simulink model "untitled"  (R2021a)
settings: Solver=VariableStepAuto  StartTime=0.0  StopTime=10  FixedStep=0.1  RelTol=0.001
libraries: simulink x1
settings Model: Creator=VTX  LastModifiedBy=VTX

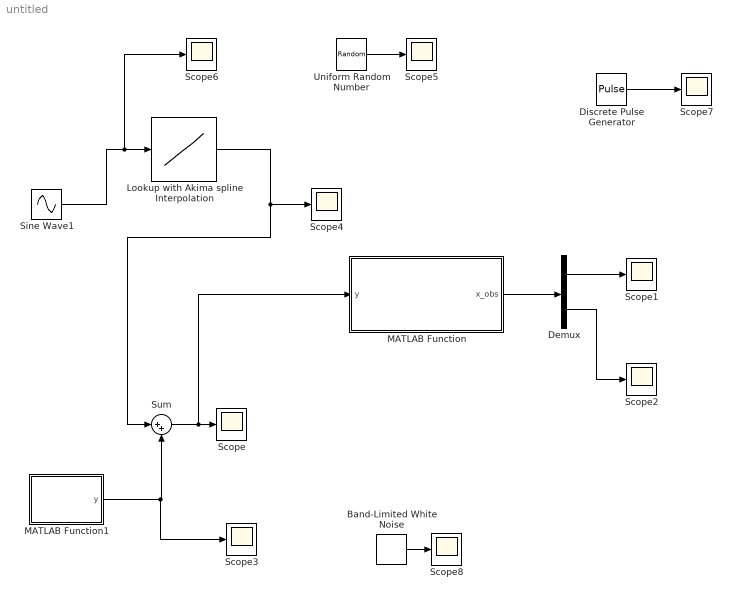
== system untitled ==
  Band-Limited White Noise : simulink/Sources/Band-Limited White Noise  Cov=[0.1]  Ts=0.1  seed=[23341]
  Demux : Demux  Outputs=2
  Discrete Pulse Generator : DiscretePulseGenerator  Period=10  PulseWidth=5  SampleTime=2
  Lookup with Akima spline Interpolation : Lookup_n-D  NumberOfTableDimensions=1  BreakpointsForDimension1=[-5:5]  Table=tanh([-5:5])  InterpMethod=Akima spline  InternalRulePriority=Speed  RndMeth=Simplest  InputSameDT=on
  MATLAB Function : MATLAB Function  TreatAsAtomicUnit=on
  MATLAB Function1 : MATLAB Function  TreatAsAtomicUnit=on
  Scope{,1..8} (9 alike) : Scope
  Sine Wave1 : Sin  SampleTime=0.1
  Sum : Sum  Inputs=|++
  Uniform Random Number : UniformRandomNumber  SampleTime=0.1
  wires:
  MATLAB Function/1(x_obs) -> Demux/1
  Demux/1 -> Scope1/1
  Demux/2 -> Scope2/1
  Sum/1 -> MATLAB Function/1(y), Scope/1
  MATLAB Function1/1(y) -> Scope3/1, Sum/2
  Sine Wave1/1 -> Scope6/1, Lookup with Akima spline Interpolation/1
  Lookup with Akima spline Interpolation/1 -> Scope4/1, Sum/1
  Uniform Random Number/1 -> Scope5/1
  Discrete Pulse Generator/1 -> Scope7/1
  Band-Limited White Noise/1 -> Scope8/1

== matlab function untitled/MATLAB Function ==
  data: y input; x_obs output
function x_obs  = fcn(y)
    x = cell(1,10);
    x{1} = zeros(2,1);

    P = cell(1,10);
    P{1} = [0.01 0;0 1];

    for j = 2:10
        %% Prediction
        x_p = [1 0.5;0 1]*x{j-1} + [0 0.5]'*(-2);
        P_p = [1 0.5;0 1]*P{j-1}*[1 0.5;0 1]' + 0.1*eye(2);
    
        %% Correction
        K = P_p*[1 0]'*inv([1 0]*P_p*[1 0]' + 0.05);
        x{j} = x_p + K*(y - [1 0]*x_p);
        P{j} = (eye(2) - K*[1 0])*P_p;
    end
    x_obs = x{10};
end

== matlab function untitled/MATLAB Function1 ==
  data: y output
function y = fcn()
    y = rand(1);
end
